simulink model "adas_top"  (R2026a)
settings: Solver=VariableStepAuto
settings Model: Creator=svvb7  LastModifiedBy=svvb7

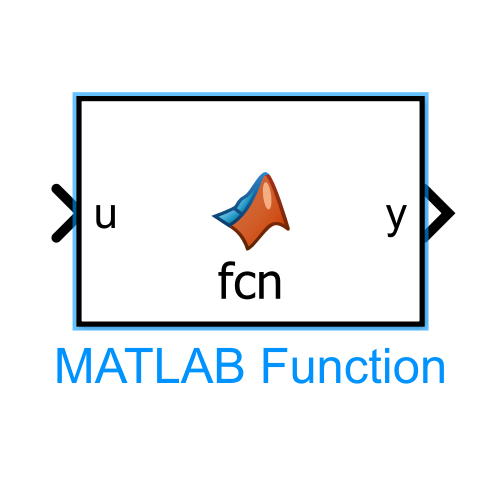
[thumbnail: Simulink's stored preview of the top-level diagram]
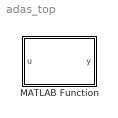
== system adas_top ==
  MATLAB Function : MATLAB Function  TreatAsAtomicUnit=on

== matlab function adas_top/MATLAB Function ==
  data: u input; y output
function y = fcn(u)
clc;
clear;
close all;

model = 'adas_top';

new_system(model);

open_system(model);

% Add blocks
add_block('simulink/Sources/In1', ...
    [model '/Video_Input']);

add_block('simulink/Math Operations/Gain', ...
    [model '/RGB2GRAY']);

add_block('simulink/Discrete/Discrete Filter', ...
    [model '/Gaussian_Filter']);

add_block('simulink/Math Operations/Add', ...
    [model '/Sobel_Filter']);

add_block('simulink/Sinks/Out1', ...
    [model '/Display_Output']);

% Connect blocks
add_line(model,'Video_Input/1','RGB2GRAY/1');

add_line(model,'RGB2GRAY/1','Gaussian_Filter/1');

add_line(model,'Gaussian_Filter/1','Sobel_Filter/1');

add_line(model,'Sobel_Filter/1','Display_Output/1');

save_system(model);

open_system(model);
